simulink model "Enhanced_BMS"  (R2024a)
settings: Solver=ode1be  StartTime=0.0  StopTime=5*3600  FixedStep=0.1  RelTol=1e-3
model workspace (MAT data in the model file):
  CC = 16
  Cell_Max_Voltage = 4.1
  I_disch = -16
  R_EOL = 0.3
  R_new = 0.05
libraries: fl_lib x31, nesl_utility x24, simulink x8, ee_lib x6, batteryecm_lib x3, slpidlib x1
(part 2 of 2)

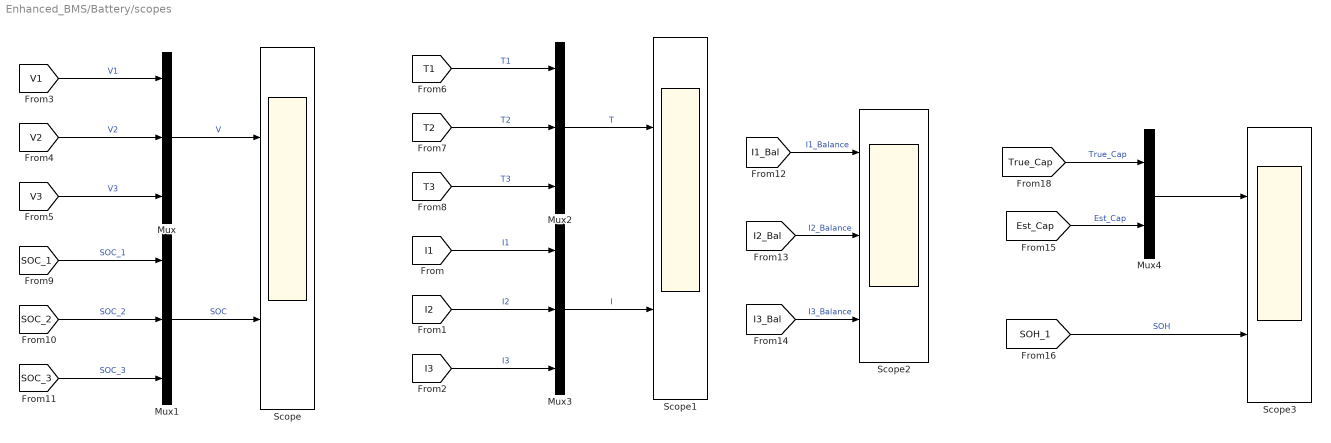
== system Enhanced_BMS/Battery/scopes ==
  Mux{,1..3} (4 alike) : Mux  Inputs=3
  Mux4 : Mux  Inputs=2
  Scope : Scope  NumInputPorts=2
  Scope1 : Scope  NumInputPorts=2
  Scope2 : Scope  NumInputPorts=3
  Scope3 : Scope  NumInputPorts=2
  wires:
  Mux/1 -> Scope/1  "V"
  Mux1/1 -> Scope/2  "SOC"
  Mux2/1 -> Scope1/1  "T"
  Mux3/1 -> Scope1/2  "I"
  [T1] -> Mux2/1  "T1"
  [T2] -> Mux2/2  "T2"
  [T3] -> Mux2/3  "T3"
  [SOC_2] -> Mux1/2  "SOC_2"
  [SOC_1] -> Mux1/1  "SOC_1"
  [SOC_3] -> Mux1/3  "SOC_3"
  [I1] -> Mux3/1  "I1"
  [I3] -> Mux3/3  "I3"
  [I2] -> Mux3/2  "I2"
  [V2] -> Mux/2  "V2"
  [V3] -> Mux/3  "V3"
  [V1] -> Mux/1  "V1"
  [I1_Bal] -> Scope2/1  "I1_Balance"
  [I3_Bal] -> Scope2/3  "I3_Balance"
  [I2_Bal] -> Scope2/2  "I2_Balance"
  [SOH_1] -> Scope3/2  "SOH"
  Mux4/1 -> Scope3/1
  [True_Cap] -> Mux4/1  "True_Cap"
  [Est_Cap] -> Mux4/2  "Est_Cap"

== system Enhanced_BMS/Battery/SOC Estimator/1RC ECM ==
  Cell1 : Subsystem
  Cell2 : Subsystem
  Cell3 : Subsystem

== system Enhanced_BMS/Battery/SOC Estimator/EKF ==
  SOC Estimation Cell 1 : Subsystem
  SOC Estimation Cell 2 : Subsystem
  SOC Estimation Cell 3 : Subsystem

== system Enhanced_BMS/Battery/SOH Estimator based on Capacit fade/SOH Estimator ==
  In1 : Inport
  Constant : Constant
  Constant1 : Constant  Value=4
  Constant2 : Constant
  Divide : Product  Inputs=*/
  Gain : Gain  Gain=100
  Sum : Sum  Inputs=|+-
  Sum1 : Sum  Inputs=|+-
  Out1 : Outport
  wires:
  Divide/1 -> Gain/1
  Constant/1 -> Sum1/2
  Sum1/1 -> Divide/2
  Constant1/1 -> Sum1/1
  Sum/1 -> Divide/1
  In1/1 -> Sum/1
  Constant2/1 -> Sum/2
  Gain/1 -> Out1/1

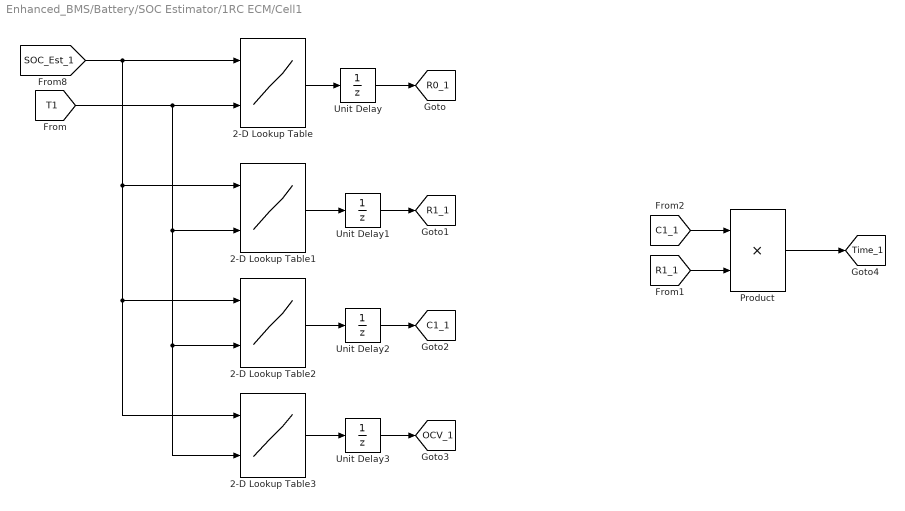
== system Enhanced_BMS/Battery/SOC Estimator/1RC ECM/Cell1 ==
  2-D Lookup Table : Lookup_n-D  BreakpointsForDimension1=[0;0.1;0.2;0.3;0.4;0.5;0.6;0.7;0.8;0.9000;1.0000]  BreakpointsForDimension2=[278.15 293.15 313.15]  Table=|  InternalRulePriority=Speed  RndMeth=Simplest
      | [0.0117    0.0085    0.0090;
      |     0.0110    0.0085    0.0090;
      |     0.0112    0.0086    0.0091;
      |     0.0114    0.0087    0.0092;
      |     0.0110    0.0084    0.0090;
      |     0.0109    0.0083    0.0088;
      |     0.0107    0.0082    0.0086;
      |     0.0107    0.0083    0.0091;
      |     0.0109    0.0086    0.0095;
      |     0.0113    0.0085    0.0089;
      |     0.0116    0.0085    0.0089]
      settings: InputPortMap=u0,u1
  2-D Lookup Table1 : Lookup_n-D  BreakpointsForDimension1=[0;0.1;0.2;0.3;0.4;0.5;0.6;0.7;0.8;0.9000;1.0000]  BreakpointsForDimension2=[278.15 293.15 313.15]  Table=|  InternalRulePriority=Speed  RndMeth=Simplest
      | [0.0109    0.0029    0.0013;
      |     0.0069    0.0024    0.0012;
      |     0.0060    0.0022    0.0011;
      |     0.0056    0.0021    0.0011;
      |     0.0052    0.0020    0.0010;
      |     0.0047    0.0016    0.0009;
      |     0.0034    0.0016    0.0010;
      |     0.0033    0.0023    0.0014;
      |     0.0033    0.0018    0.0011;
      |     0.0028    0.0017    0.0011;
      |     0.0026    0.0016    0.0010]
      settings: InputPortMap=u0,u1
  2-D Lookup Table2 : Lookup_n-D  BreakpointsForDimension1=[0;0.1;0.2;0.3;0.4;0.5;0.6;0.7;0.8;0.9000;1.0000]  BreakpointsForDimension2=[278.15 293.15 313.15]  Table=|  InternalRulePriority=Speed  RndMeth=Simplest
      | [
      |     1917, 12414, 30615;
      |     4652, 18875, 33000;
      |     3533, 12864, 40000;
      |     23286, 4810, 47545;
      |     20000, 3100, 36500;
      |     1745, 18750, 26333;
      |     18029, 33625, 48300;
      |     15030, 53696, 38143;
      |     12242, 18389, 26727;
      |     10000, 19882, 16727;
      |     9038, 23375, 3600
      | ];
      settings: InputPortMap=u0,u1
  2-D Lookup Table3 : Lookup_n-D  BreakpointsForDimension1=[0;0.1;0.2;0.3;0.4;0.5;0.6;0.7;0.8;0.9000;1.0000]  BreakpointsForDimension2=[278.15 293.15 313.15]  Table=|  InternalRulePriority=Speed  RndMeth=Simplest
      | [3.4966    3.5057    3.5148;
      |     3.5519    3.5660    3.5653;
      |     3.5813    3.5911    3.5999;
      |     3.6183    3.6337    3.6402;
      |     3.6871    3.6921    3.6993;
      |     3.7066    3.7127    3.7213;
      |     3.7611    3.7665    3.7922;
      |     3.8111    3.8531    3.8971;
      |     3.9131    3.9259    3.9376;
      |     4.0748    4.0777    4.0821;
      |     4.1923    4.1928    4.1930]
      settings: InputPortMap=u0,u1
  Product : Product
  Unit Delay : UnitDelay  InitialCondition=0.0084  SampleTime=-1  HasFrameUpgradeWarning=on
  Unit Delay1 : UnitDelay  InitialCondition=0.0020  SampleTime=-1  HasFrameUpgradeWarning=on
  Unit Delay2 : UnitDelay  InitialCondition=0.0310  SampleTime=-1  HasFrameUpgradeWarning=on
  Unit Delay3 : UnitDelay  InitialCondition=3.6921  SampleTime=-1  HasFrameUpgradeWarning=on
  tag scope: C1_1=global, OCV_1=global, R0_1=global, R1_1=global, Time_1=global
  wires:
  2-D Lookup Table/1 -> Unit Delay/1
  2-D Lookup Table1/1 -> Unit Delay1/1
  2-D Lookup Table2/1 -> Unit Delay2/1
  2-D Lookup Table3/1 -> Unit Delay3/1
  [SOC_Est_1] -> 2-D Lookup Table3/1, 2-D Lookup Table2/1, 2-D Lookup Table1/1, 2-D Lookup Table/1
  [T1] -> 2-D Lookup Table3/2, 2-D Lookup Table2/2, 2-D Lookup Table1/2, 2-D Lookup Table/2
  Unit Delay/1 -> [R0_1]
  Unit Delay1/1 -> [R1_1]
  Unit Delay2/1 -> [C1_1]
  Unit Delay3/1 -> [OCV_1]
  [R1_1] -> Product/2
  [C1_1] -> Product/1
  Product/1 -> [Time_1]

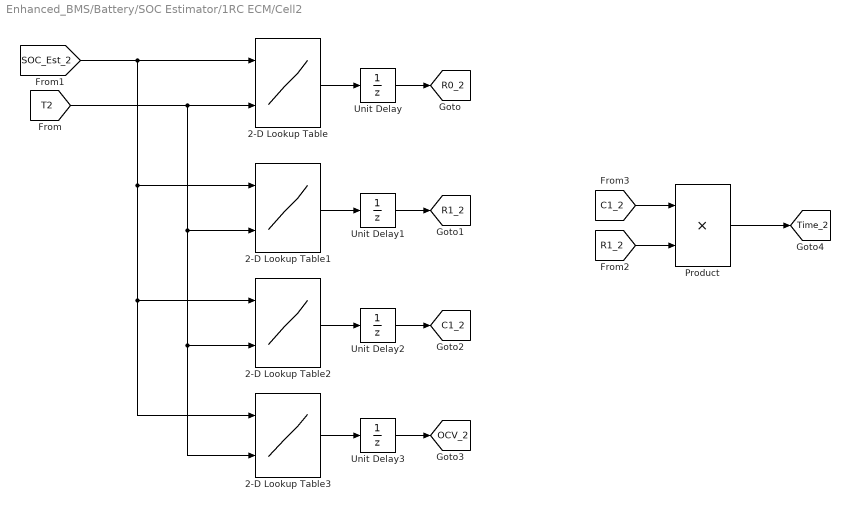
== system Enhanced_BMS/Battery/SOC Estimator/1RC ECM/Cell2 ==
  2-D Lookup Table : Lookup_n-D  BreakpointsForDimension1=[0;0.1;0.2;0.3;0.4;0.5;0.6;0.7;0.8;0.9000;1.0000]  BreakpointsForDimension2=[278.15 293.15 313.15]  Table=|  InternalRulePriority=Speed  RndMeth=Simplest
      | [0.0113    0.0091    0.0083;
      |     0.0108    0.0079    0.0092;
      |     0.0111    0.0083    0.0094;
      |     0.0110    0.0090    0.0096;
      |     0.0108    0.0080    0.0087;
      |     0.0107    0.0085    0.0091;
      |     0.0106    0.0081    0.0087;
      |     0.0106    0.0082    0.0090;
      |     0.0111    0.0084    0.0093;
      |     0.0111    0.0082    0.0090;
      |     0.0115    0.0084    0.0093]
      settings: InputPortMap=u0,u1
  2-D Lookup Table1 : Lookup_n-D  BreakpointsForDimension1=[0;0.1;0.2;0.3;0.4;0.5;0.6;0.7;0.8;0.9000;1.0000]  BreakpointsForDimension2=[278.15 293.15 313.15]  Table=|  InternalRulePriority=Speed  RndMeth=Simplest
      | [0.0107    0.0028    0.0012;
      |                0.0070    0.0023    0.0011;
      |                0.0061    0.0021    0.0012;
      |                0.0057    0.0022    0.0010;
      |                0.0051    0.0021    0.0010;
      |                0.0048    0.0017    0.0009;
      |                0.0035    0.0017    0.0010;
      |                0.0034    0.0023    0.0015;
      |                0.0033    0.0018    0.0011;
      |                0.0027    0.0016    0.0011;
      |                0.0025    0.0017    0.0010]
      settings: InputPortMap=u0,u1
  2-D Lookup Table2 : Lookup_n-D  BreakpointsForDimension1=[0;0.1;0.2;0.3;0.4;0.5;0.6;0.7;0.8;0.9000;1.0000]  BreakpointsForDimension2=[278.15 293.15 313.15]  Table=|  InternalRulePriority=Speed  RndMeth=Simplest
      | [
      |     2140.0, 13357.0, 34500.0;
      |     47860.0, 20391.0, 35455.0;
      |     35740.0, 13762.0, 37083.0;
      |     23018.0, 4909.0, 51200.0;
      |     20216.0, 3238.0, 36700.0;
      |     16670.0, 18706.0, 24667.0;
      |     17743.0, 32588.0, 49300.0;
      |     14382.0, 53783.0, 35400.0;
      |     12455.0, 18222.0, 27364.0;
      |     10630.0, 21688.0, 17636.0;
      |     9760.0, 22118.0, 2500.0
      | ];
      settings: InputPortMap=u0,u1
  2-D Lookup Table3 : Lookup_n-D  BreakpointsForDimension1=[0;0.1;0.2;0.3;0.4;0.5;0.6;0.7;0.8;0.9000;1.0000]  BreakpointsForDimension2=[278.15 293.15 313.15]  Table=|  InternalRulePriority=Speed  RndMeth=Simplest
      | [3.3982    3.4675    3.5113;
      |     3.4661    3.4887    3.5583;
      |     3.5049    3.5349    3.5691;
      |     3.6028    3.6097    3.6454;
      |     3.6308    3.6507    3.6665;
      |     3.6894    3.7048    3.7223;
      |     3.7552    3.7841    3.8085;
      |     3.8036    3.8479    3.8945;
      |     3.9046    3.9305    3.9620;
      |     4.0752    4.0786    4.1127;
      |     4.1734    4.1926    4.2048]
      settings: InputPortMap=u0,u1
  Product : Product
  Unit Delay{,1..3} (4 alike) : UnitDelay  InitialCondition=0.0084  SampleTime=-1  HasFrameUpgradeWarning=on
  tag scope: C1_2=global, OCV_2=global, R0_2=global, R1_2=global, Time_2=global
  wires:
  2-D Lookup Table/1 -> Unit Delay/1
  2-D Lookup Table1/1 -> Unit Delay1/1
  2-D Lookup Table2/1 -> Unit Delay2/1
  2-D Lookup Table3/1 -> Unit Delay3/1
  [T2] -> 2-D Lookup Table3/2, 2-D Lookup Table2/2, 2-D Lookup Table1/2, 2-D Lookup Table/2
  [SOC_Est_2] -> 2-D Lookup Table3/1, 2-D Lookup Table2/1, 2-D Lookup Table1/1, 2-D Lookup Table/1
  Unit Delay/1 -> [R0_2]
  Unit Delay1/1 -> [R1_2]
  Unit Delay2/1 -> [C1_2]
  Unit Delay3/1 -> [OCV_2]
  Product/1 -> [Time_2]
  [R1_2] -> Product/2
  [C1_2] -> Product/1

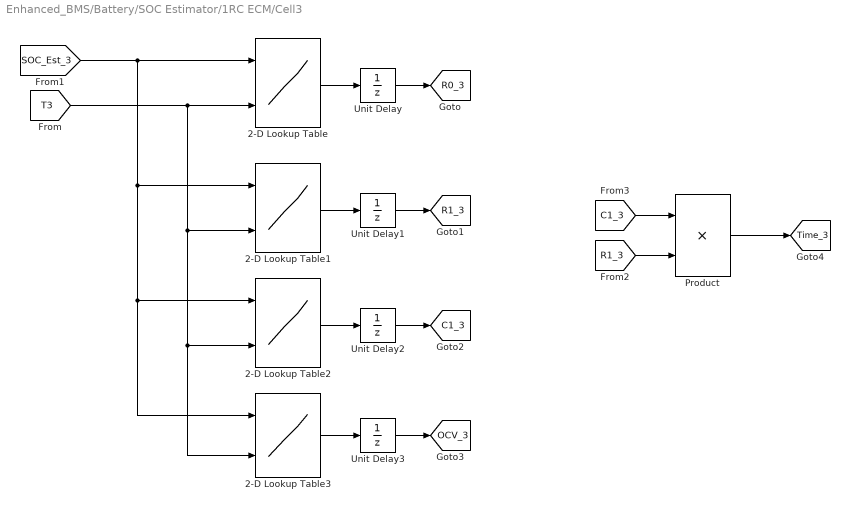
== system Enhanced_BMS/Battery/SOC Estimator/1RC ECM/Cell3 ==
  2-D Lookup Table : Lookup_n-D  BreakpointsForDimension1=[0;0.1;0.2;0.3;0.4;0.5;0.6;0.7;0.8;0.9000;1.0000]  BreakpointsForDimension2=[278.15 293.15 313.15]  Table=|  InternalRulePriority=Speed  RndMeth=Simplest
      | [0.0111    0.0088    0.0094;
      |     0.0109    0.0083    0.0091;
      |     0.0113    0.0087    0.0092;
      |     0.0115    0.0089    0.0090;
      |     0.0112    0.0083    0.0092;
      |     0.0108    0.0082    0.0085;
      |     0.0109    0.0080    0.0088;
      |     0.0108    0.0085    0.0092;
      |     0.0110    0.0087    0.0095;
      |     0.0110    0.0084    0.0090;
      |     0.0112    0.0085    0.0092]
      settings: InputPortMap=u0,u1
  2-D Lookup Table1 : Lookup_n-D  BreakpointsForDimension1=[0;0.1;0.2;0.3;0.4;0.5;0.6;0.7;0.8;0.9000;1.0000]  BreakpointsForDimension2=[278.15 293.15 313.15]  Table=|  InternalRulePriority=Speed  RndMeth=Simplest
      | [0.0108    0.0029    0.0014;
      |     0.0071    0.0025    0.0013;
      |     0.0062    0.0023    0.0012;
      |     0.0058    0.0022    0.0011;
      |     0.0053    0.0020    0.0011;
      |     0.0049    0.0017    0.0008;
      |     0.0034    0.0016    0.0011;
      |     0.0032    0.0024    0.0015;
      |     0.0034    0.0019    0.0012;
      |     0.0029    0.0018    0.0012;
      |     0.0027    0.0016    0.0011]
      settings: InputPortMap=u0,u1
  2-D Lookup Table2 : Lookup_n-D  BreakpointsForDimension1=[0;0.1;0.2;0.3;0.4;0.5;0.6;0.7;0.8;0.9000;1.0000]  BreakpointsForDimension2=[278.15 293.15 313.15]  Table=|  InternalRulePriority=Speed  RndMeth=Simplest
      | [
      |     2481.0, 14517.0, 31143.0;
      |     49440.0, 18680.0, 29154.0;
      |     34030.0, 12000.0, 37833.0;
      |     22397.0, 5227.0, 48091.0;
      |     19547.0, 3000.0, 33909.0;
      |     14490.0, 17706.0, 26625.0;
      |     18647.0, 32875.0, 44091.0;
      |     15750.0, 50792.0, 35200.0;
      |     12294.0, 17368.0, 25250.0;
      |     98280.0, 18944.0, 14917.0;
      |     89260.0, 24188.0, 2455.0
      | ];
      settings: InputPortMap=u0,u1
  2-D Lookup Table3 : Lookup_n-D  BreakpointsForDimension1=[0;0.1;0.2;0.3;0.4;0.5;0.6;0.7;0.8;0.9000;1.0000]  BreakpointsForDimension2=[278.15 293.15 313.15]  Table=|  InternalRulePriority=Speed  RndMeth=Simplest
      | [3.5401    3.5396    3.5774;
      |     3.5358    3.5420    3.5681;
      |     3.5927    3.5929    3.6060;
      |     3.6439    3.6419    3.6703;
      |     3.6918    3.7065    3.7267;
      |     3.7452    3.7613    3.7676;
      |     3.8012    3.8302    3.8439;
      |     3.8387    3.8762    3.9140;
      |     3.9398    3.9668    3.9903;
      |     4.1102    4.1221    4.1420;
      |     4.1742    4.2065    4.2399]
      settings: InputPortMap=u0,u1
  Product : Product
  Unit Delay{,1..3} (4 alike) : UnitDelay  InitialCondition=0.0084  SampleTime=-1  HasFrameUpgradeWarning=on
  tag scope: C1_3=global, OCV_3=global, R0_3=global, R1_3=global, Time_3=global
  wires:
  2-D Lookup Table/1 -> Unit Delay/1
  2-D Lookup Table1/1 -> Unit Delay1/1
  2-D Lookup Table2/1 -> Unit Delay2/1
  2-D Lookup Table3/1 -> Unit Delay3/1
  [T3] -> 2-D Lookup Table3/2, 2-D Lookup Table2/2, 2-D Lookup Table1/2, 2-D Lookup Table/2
  [SOC_Est_3] -> 2-D Lookup Table3/1, 2-D Lookup Table2/1, 2-D Lookup Table1/1, 2-D Lookup Table/1
  Unit Delay/1 -> [R0_3]
  Unit Delay1/1 -> [R1_3]
  Unit Delay2/1 -> [C1_3]
  Unit Delay3/1 -> [OCV_3]
  Product/1 -> [Time_3]
  [R1_3] -> Product/2
  [C1_3] -> Product/1

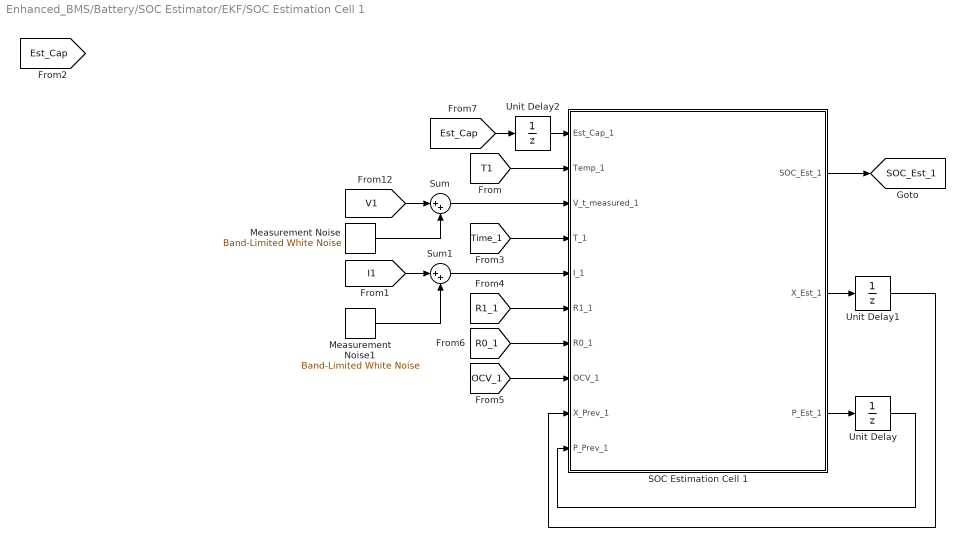
== system Enhanced_BMS/Battery/SOC Estimator/EKF/SOC Estimation Cell 1 ==
  Measurement Noise : simulink/Sources/Band-Limited White Noise  Cov=1e-2  Ts=0.1  seed=1234
  Measurement Noise1 : simulink/Sources/Band-Limited White Noise  Cov=1e-2  Ts=0.1  seed=1234
  SOC Estimation Cell 1 : MATLAB Function  TreatAsAtomicUnit=on
  Sum : Sum  Inputs=|++
  Sum1 : Sum  Inputs=|++
  Unit Delay : UnitDelay  InitialCondition=[0.02 0 ; 0 0.01]  SampleTime=-1  HasFrameUpgradeWarning=on
  Unit Delay1 : UnitDelay  InitialCondition=[0.4;0]  SampleTime=-1  HasFrameUpgradeWarning=on
  Unit Delay2 : UnitDelay  InitialCondition=4  SampleTime=-1  HasFrameUpgradeWarning=on
  tag scope: SOC_Est_1=global
  wires:
  Measurement Noise/1 -> Sum/2
  [V1] -> Sum/1
  [T1] -> SOC Estimation Cell 1/2(Temp_1)
  Sum/1 -> SOC Estimation Cell 1/3(V_t_measured_1)
  SOC Estimation Cell 1/2(X_Est_1) -> Unit Delay1/1
  SOC Estimation Cell 1/3(P_Est_1) -> Unit Delay/1
  Unit Delay/1 -> SOC Estimation Cell 1/10(P_Prev_1)
  Unit Delay1/1 -> SOC Estimation Cell 1/9(X_Prev_1)
  [R1_1] -> SOC Estimation Cell 1/6(R1_1)
  [OCV_1] -> SOC Estimation Cell 1/8(OCV_1)
  [R0_1] -> SOC Estimation Cell 1/7(R0_1)
  SOC Estimation Cell 1/1(SOC_Est_1) -> [SOC_Est_1]
  Measurement Noise1/1 -> Sum1/2
  [I1] -> Sum1/1
  [Time_1] -> SOC Estimation Cell 1/4(T_1)
  Sum1/1 -> SOC Estimation Cell 1/5(I_1)
  [Est_Cap] -> Unit Delay2/1
  Unit Delay2/1 -> SOC Estimation Cell 1/1(Est_Cap_1)

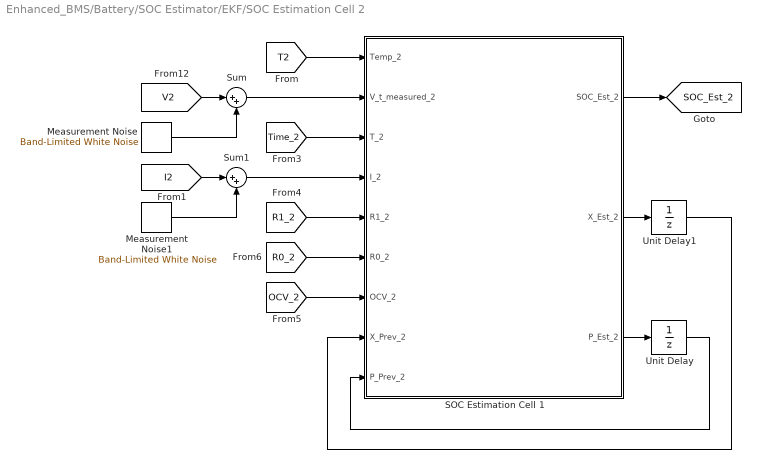
== system Enhanced_BMS/Battery/SOC Estimator/EKF/SOC Estimation Cell 2 ==
  Measurement Noise : simulink/Sources/Band-Limited White Noise  Cov=1e-2  Ts=0.1  seed=1234
  Measurement Noise1 : simulink/Sources/Band-Limited White Noise  Cov=1e-2  Ts=0.1  seed=1234
  SOC Estimation Cell 1 : MATLAB Function  TreatAsAtomicUnit=on
  Sum : Sum  Inputs=|++
  Sum1 : Sum  Inputs=|++
  Unit Delay : UnitDelay  InitialCondition=[0.02 0 ; 0 0.01]  SampleTime=-1  HasFrameUpgradeWarning=on
  Unit Delay1 : UnitDelay  InitialCondition=[0.4;0]  SampleTime=-1  HasFrameUpgradeWarning=on
  tag scope: SOC_Est_2=global
  wires:
  SOC Estimation Cell 1/1(SOC_Est_2) -> [SOC_Est_2]
  [R1_2] -> SOC Estimation Cell 1/5(R1_2)
  [R0_2] -> SOC Estimation Cell 1/6(R0_2)
  [T2] -> SOC Estimation Cell 1/1(Temp_2)
  [Time_2] -> SOC Estimation Cell 1/3(T_2)
  [OCV_2] -> SOC Estimation Cell 1/7(OCV_2)
  Unit Delay1/1 -> SOC Estimation Cell 1/8(X_Prev_2)
  SOC Estimation Cell 1/2(X_Est_2) -> Unit Delay1/1
  Sum/1 -> SOC Estimation Cell 1/2(V_t_measured_2)
  Unit Delay/1 -> SOC Estimation Cell 1/9(P_Prev_2)
  [V2] -> Sum/1
  SOC Estimation Cell 1/3(P_Est_2) -> Unit Delay/1
  Measurement Noise/1 -> Sum/2
  Sum1/1 -> SOC Estimation Cell 1/4(I_2)
  Measurement Noise1/1 -> Sum1/2
  [I2] -> Sum1/1

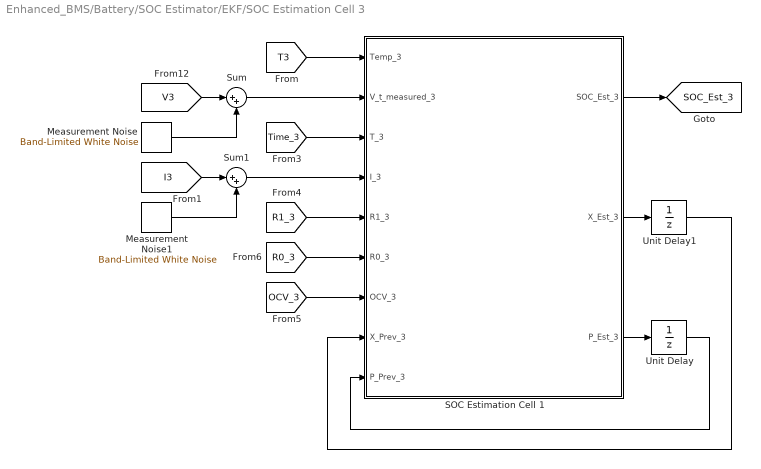
== system Enhanced_BMS/Battery/SOC Estimator/EKF/SOC Estimation Cell 3 ==
  Measurement Noise : simulink/Sources/Band-Limited White Noise  Cov=1e-2  Ts=0.1  seed=1234
  Measurement Noise1 : simulink/Sources/Band-Limited White Noise  Cov=1e-2  Ts=0.1  seed=1234
  SOC Estimation Cell 1 : MATLAB Function  TreatAsAtomicUnit=on
  Sum : Sum  Inputs=|++
  Sum1 : Sum  Inputs=|++
  Unit Delay : UnitDelay  InitialCondition=[0.02 0 ; 0 0.01]  SampleTime=-1  HasFrameUpgradeWarning=on
  Unit Delay1 : UnitDelay  InitialCondition=[0.4;0]  SampleTime=-1  HasFrameUpgradeWarning=on
  tag scope: SOC_Est_3=global
  wires:
  SOC Estimation Cell 1/1(SOC_Est_3) -> [SOC_Est_3]
  [R1_3] -> SOC Estimation Cell 1/5(R1_3)
  [R0_3] -> SOC Estimation Cell 1/6(R0_3)
  [T3] -> SOC Estimation Cell 1/1(Temp_3)
  [Time_3] -> SOC Estimation Cell 1/3(T_3)
  [OCV_3] -> SOC Estimation Cell 1/7(OCV_3)
  Unit Delay1/1 -> SOC Estimation Cell 1/8(X_Prev_3)
  SOC Estimation Cell 1/2(X_Est_3) -> Unit Delay1/1
  Sum/1 -> SOC Estimation Cell 1/2(V_t_measured_3)
  Unit Delay/1 -> SOC Estimation Cell 1/9(P_Prev_3)
  [V3] -> Sum/1
  SOC Estimation Cell 1/3(P_Est_3) -> Unit Delay/1
  Measurement Noise/1 -> Sum/2
  Measurement Noise1/1 -> Sum1/2
  [I3] -> Sum1/1
  Sum1/1 -> SOC Estimation Cell 1/4(I_3)

== matlab function Enhanced_BMS/Battery/SOH Estimator based on Capacit fade/Capacity Estimator ==
  data: Prev_Est_Cap input; I_C1 input; SOC1 input; SOC2 input; Prev_Est_P input; Est_Cap output; Est_P output
function [Est_Cap,Est_P] = Capcity_Estimator(Prev_Est_Cap,I_C1,SOC1,SOC2,Prev_Est_P)

% initialization
A = 1;
R = 1.5e-3;
Q = 2.1e-3;

% Prediction
Pred_Cap = A * Prev_Est_Cap;
Pred_P = A * Prev_Est_P * A + Q;

% Correction
H = -(I_C1*0.1) / (((Prev_Est_Cap)^2)*3600);

Y_error =  (SOC2 - SOC1) - (H * Pred_Cap);

K = Pred_P*H'/(H*Pred_P*H'+R);

Est_Cap = Pred_Cap + K*Y_error;
Est_P = (1 - K*H)*Pred_P;

end

== stateflow chart Enhanced_BMS/Chart ==
  state wait
  state CHG
    entry:
    Mode = 2;
  state DISCH
    entry:
    Mode = 1;
  (default) -> wait
  wait -> (junction 11) [order 1] : [SOC_Max>0.5]
  (junction 11) -> DISCH
  wait -> CHG [order 2] : [SOC_Max<0.5]
  CHG -> DISCH : [SOC_Max>0.9 || after(7000,sec)]
  DISCH -> CHG : [SOC_Min<0.2]
  data: SOC_Max input; Mode output; SOC_Min input

== matlab function Enhanced_BMS/Battery/SOC Estimator/EKF/SOC Estimation Cell 1/SOC Estimation Cell 1 ==
  data: Est_Cap_1 input; SOC_Est_1 output; Temp_1 input; V_t_measured_1 input; T_1 input; I_1 input; R1_1 input; R0_1 input; OCV_1 input; X_Est_1 output; P_Est_1 output; X_Prev_1 input; P_Prev_1 input
function [SOC_Est_1,X_Est_1,P_Est_1] = EKF_1(Est_Cap_1,Temp_1,V_t_measured_1,T_1,I_1,R1_1,R0_1,OCV_1, X_Prev_1,P_Prev_1)
% initialization
A_1 = [1 0 ; 0 exp(-0.1/T_1)];
B_1 = [-0.1/(Est_Cap_1*3600); R1_1*(1-exp(-0.1/T_1))];
Q_1 = [1e-6 0;0 1e-6];
R_1 = 3.3;

% Prediction
X_Current_1 = A_1*X_Prev_1 + B_1*I_1;
P_Current_1 = A_1*P_Prev_1*A_1'+Q_1;
SOC_current_1 = X_Current_1(1);

if (278.15 <= Temp_1) && (Temp_1 < 293.15)
dOCV_1_dSOC = 1.1060 - 2*8.8431*(SOC_current_1) + 3*41.1474*(SOC_current_1)^2 - 4*86.4016*(SOC_current_1)^3+5*83.0540*(SOC_current_1)^4 - 6*29.3668*(SOC_current_1)^5;
elseif (293.15 <= Temp_1) && (Temp_1 < 313.15)
dOCV_1_dSOC = 0.9211 - 2*5.4454*(SOC_current_1) + 3*23.0563*(SOC_current_1)^2 - 4*46.4109*(SOC_current_1)^3+5*44.1992*(SOC_current_1)^4 - 6*15.6332*(SOC_current_1)^5;
elseif Temp_1 >= 313.15
dOCV_1_dSOC = 0.6001 - 2*1.5306*(SOC_current_1) + 3*4.9231*(SOC_current_1)^2 - 4*7.7784*(SOC_current_1)^3+5*6.7360*(SOC_current_1)^4 - 6*2.2704*(SOC_current_1)^5;
else
    error("undefined")
end

H_1 = [dOCV_1_dSOC -1];

% Correction
K_1 = (P_Current_1*H_1')/(H_1*P_Current_1*H_1'+R_1);
X_Est_1 = X_Current_1 + K_1*(V_t_measured_1 - (OCV_1 - X_Current_1(2) - I_1*R0_1));
P_Est_1 = (eye(2) - K_1*H_1)*P_Current_1;
SOC_Est_1 = X_Est_1(1);
end

== matlab function Enhanced_BMS/Battery/SOC Estimator/EKF/SOC Estimation Cell 2/SOC Estimation Cell 1 ==
  data: SOC_Est_2 output; Temp_2 input; V_t_measured_2 input; T_2 input; I_2 input; R1_2 input; R0_2 input; OCV_2 input; X_Est_2 output; P_Est_2 output; X_Prev_2 input; P_Prev_2 input
function [SOC_Est_2,X_Est_2,P_Est_2] = EKF_2(Temp_2,V_t_measured_2,T_2,I_2,R1_2,R0_2,OCV_2, X_Prev_2,P_Prev_2)
% initialization
A_2 = [1 0 ; 0 exp(-0.1/T_2)];
B_2 = [-0.1/(4*3600); R1_2*(1-exp(-0.1/T_2))];
Q_2 = [1e-6 0;0 1e-6];
R_2 = 3.3;
% Prediction
X_Current_2 = A_2*X_Prev_2 + B_2*I_2;
P_Current_2 = A_2*P_Prev_2*A_2'+Q_2;
SOC_current_2 = X_Current_2(1);

if (278.15 <= Temp_2) && (Temp_2 < 293.15)
dOCV_2_dSOC = 1.1060 - 2*8.8431*(SOC_current_2) + 3*41.1474*(SOC_current_2)^2 - 4*86.4016*(SOC_current_2)^3+5*83.0540*(SOC_current_2)^4 - 6*29.3668*(SOC_current_2)^5;
elseif (293.15 <= Temp_2) && (Temp_2 < 313.15)
dOCV_2_dSOC = 0.9211 - 2*5.4454*(SOC_current_2) + 3*23.0563*(SOC_current_2)^2 - 4*46.4109*(SOC_current_2)^3+5*44.1992*(SOC_current_2)^4 - 6*15.6332*(SOC_current_2)^5;
elseif Temp_2 >= 313.15
dOCV_2_dSOC = 0.6001 - 2*1.5306*(SOC_current_2) + 3*4.9231*(SOC_current_2)^2 - 4*7.7784*(SOC_current_2)^3+5*6.7360*(SOC_current_2)^4 - 6*2.2704*(SOC_current_2)^5;
else
    error("undefined")
end

H_2 = [dOCV_2_dSOC -1];

% Correction
K_2 = (P_Current_2*H_2')/(H_2*P_Current_2*H_2'+R_2);
X_Est_2 = X_Current_2 + K_2*(V_t_measured_2 - (OCV_2 - X_Current_2(2) - I_2*R0_2));
P_Est_2 = (eye(2) - K_2*H_2)*P_Current_2;
SOC_Est_2 = X_Est_2(1);
end

== matlab function Enhanced_BMS/Battery/SOC Estimator/EKF/SOC Estimation Cell 3/SOC Estimation Cell 1 ==
  data: SOC_Est_3 output; Temp_3 input; V_t_measured_3 input; T_3 input; I_3 input; R1_3 input; R0_3 input; OCV_3 input; X_Est_3 output; P_Est_3 output; X_Prev_3 input; P_Prev_3 input
function [SOC_Est_3,X_Est_3,P_Est_3] = EKF_3(Temp_3,V_t_measured_3,T_3,I_3,R1_3,R0_3,OCV_3, X_Prev_3,P_Prev_3)
% initialization
A_3 = [1 0 ; 0 exp(-0.1/T_3)];
B_3 = [-0.1/(4*3600); R1_3*(1-exp(-0.1/T_3))];
Q_3 = [1e-6 0;0 1e-6];
R_3 = 3.3;
% Prediction
X_Current_3 = A_3*X_Prev_3 + B_3*I_3;
P_Current_3 = A_3*P_Prev_3*A_3'+Q_3;
SOC_current_3 = X_Current_3(1);

if (278.15 <= Temp_3) && (Temp_3 < 293.15)
dOCV_3_dSOC = 1.1060 - 2*8.8431*(SOC_current_3) + 3*41.1474*(SOC_current_3)^2 - 4*86.4016*(SOC_current_3)^3+5*83.0540*(SOC_current_3)^4 - 6*29.3668*(SOC_current_3)^5;
elseif (293.15 <= Temp_3) && (Temp_3 < 313.15)
dOCV_3_dSOC = 0.9211 - 2*5.4454*(SOC_current_3) + 3*23.0563*(SOC_current_3)^2 - 4*46.4109*(SOC_current_3)^3+5*44.1992*(SOC_current_3)^4 - 6*15.6332*(SOC_current_3)^5;
elseif Temp_3 >= 313.15
dOCV_3_dSOC = 0.6001 - 2*1.5306*(SOC_current_3) + 3*4.9231*(SOC_current_3)^2 - 4*7.7784*(SOC_current_3)^3+5*6.7360*(SOC_current_3)^4 - 6*2.2704*(SOC_current_3)^5;
else
    error("undefined")
end

H_3 = [dOCV_3_dSOC -1];

% Correction
K_3 = (P_Current_3*H_3')/(H_3*P_Current_3*H_3'+R_3);
X_Est_3 = X_Current_3 + K_3*(V_t_measured_3 - (OCV_3 - X_Current_3(2) - I_3*R0_3));
P_Est_3 = (eye(2) - K_3*H_3)*P_Current_3;
SOC_Est_3 = X_Est_3(1);
end

== stateflow chart Enhanced_BMS/Battery/Balancing Algorithm ==
  state start
    entry:
    S1 = 0;
    S2 = 0;
    S3 = 0;
  state finish
    entry:
    S1 = 0;
    S2 = 0;
    S3 = 0;
  state Balancing
    during:
    S = order(V1,V2,V3);
    state wait
      wait -> (junction 29)
    state cell3_Lowest
      entry:
      S1 = 1; S3 = 1;
      S5 = 0;S6 = 0;
      S2 = 0;S4 = 0;
      during:
      if (V1 - V2) > 0.02
      S2 = 1;
      elseif (V2 - V1) > 0.02
      S4 = 1;
      end
      exit:
      S1 = 0; S2 = 0;
      S3 = 0; S4 = 0;
      S5 = 0; S6 = 0;
      S = order(V1,V2,V3);
    state cell2_Lowest
      entry:
      S1 = 1; S5 = 1;
      S3 = 0;S4 = 0;
      S2 = 0;S6 = 0;
      during:
      if (V1 - V3) > 0.02
      S2 = 1;
      elseif (V3 - V1) > 0.02
      S4 = 6;
      end
      exit:
      S1 = 0; S2 = 0;
      S3 = 0; S4 = 0;
      S5 = 0; S6 = 0;
      S = order(V1,V2,V3);
    state cell1_Lowest
      entry:
      S3 = 1; S5 = 1;
      S1 = 0;S2 = 0;
      S4 = 0;S6 = 0;
      during:
      if (V2 - V3) > 0.02
      S4 = 1;
      elseif (V3 - V2) > 0.02
      S6 = 1;
      end
      exit:
      S1 = 0; S2 = 0;
      S3 = 0; S4 = 0;
      S5 = 0; S6 = 0;
      S = order(V1,V2,V3);
    (default) -> wait
    (junction 29) -> (junction 32) [order 3] : [S(1)==3]
    (junction 29) -> (junction 60) [order 1] : [S(1)==3]
    (junction 29) -> (junction 34) [order 2] : [S(1)==2]
    (junction 32) -> cell1_Lowest
    (junction 60) -> cell3_Lowest
    (junction 34) -> cell2_Lowest
    cell2_Lowest -> cell1_Lowest [order 2] : [S(1)==1]
    cell3_Lowest -> cell2_Lowest [order 1] : [S(1)==2]
    cell2_Lowest -> cell3_Lowest [order 1] : [S(1)==3]
    cell1_Lowest -> cell2_Lowest [order 1] : [S(1)==2]
    (junction 54) -> cell3_Lowest
    cell3_Lowest -> (junction 47) [order 2]
    (junction 49) -> cell1_Lowest
    cell1_Lowest -> (junction 52) [order 2]
    (junction 47) -> (junction 49) : [S(1)==1]
    (junction 52) -> (junction 54) : [S(1)==3]
  (default) -> start
  start -> Balancing : [abs(max([V1,V2,V3])-min([V1,V2,V3])) > Threshold]
  finish -> Balancing : [abs(max([V1,V2,V3])-min([V1,V2,V3])) > Threshold]
  Balancing -> finish : [abs(max([V1,V2,V3])-min([V1,V2,V3])) < Threshold]
  data: A function_input; B function_input; C function_input; P function_output; V1 input; V2 input; V3 input; S1 output; S2 output; S3 output; Threshold local =0.02; S local; S4 output; S5 output; S6 output
  function P = order(A,B,C):
    | function P = order(A,B,C)
    | [~,P] = sort([A,B,C],'ascend');
    | end
